simulink subsystem "Speed_PI_D"  (R2022b)
settings: Solver=VariableStepAuto  StartTime=0.0  StopTime=10.0  RelTol=1e-3
undefined symbols (not defined in the file or in its folder): conv, DiscIntNeverNeededParam, motor, Ri, Rw, sat, uc
settings Model: Creator=gotta  LastModifiedBy=gotta

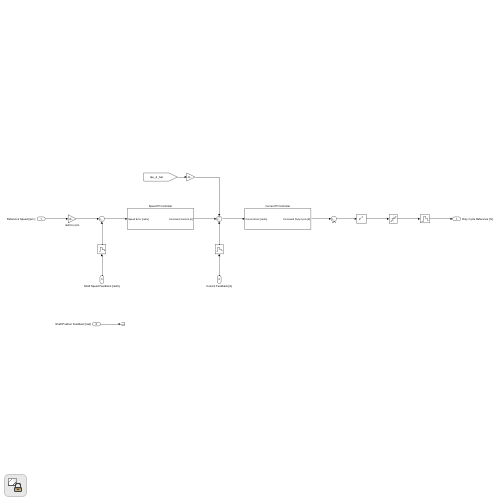
[thumbnail: Simulink's stored preview of the top-level diagram]
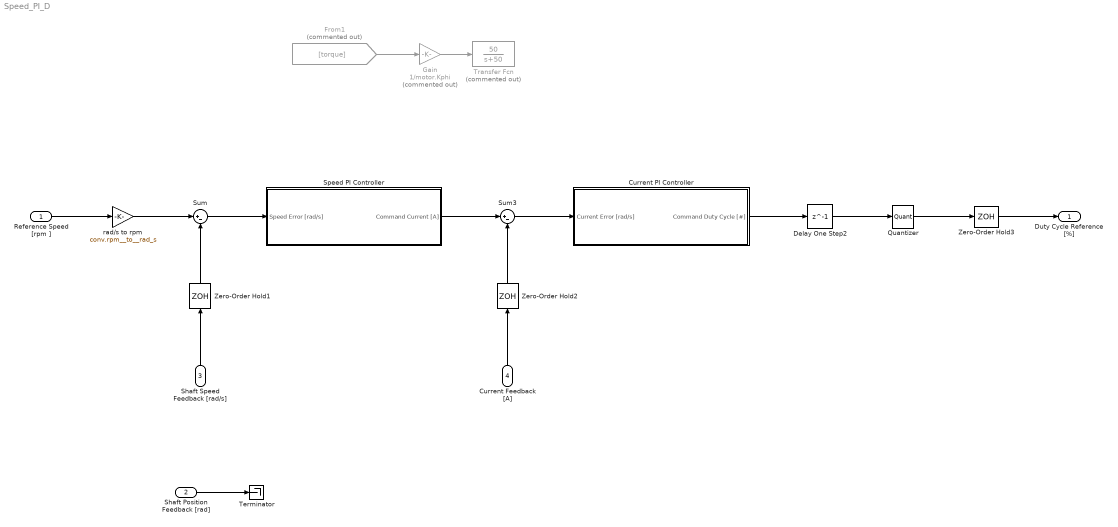
== system Speed_PI_D ==
  Reference Speed [rpm ] : Inport
  Shaft Position Feedback [rad] : Inport  Port=2
  Shaft Speed Feedback [rad/s] : Inport  Port=3
  Current Feedback [A] : Inport  Port=4
  Current PI Controller : Subsystem
  Delay One Step2 : Delay  DelayLength=1
  From1 : From  Commented=on  GotoTag=torque
  Gain : Gain  Commented=on  Gain=1/motor.Kphi
  Quantizer : Quantizer  QuantizationInterval=uc.d_step
  Speed PI Controller : Subsystem
  Sum : Sum  Inputs=|+-
  Sum3 : Sum  Inputs=|+-
  Terminator : Terminator
  Transfer Fcn : TransferFcn  Commented=on  Numerator=[50]  Denominator=[1 50]
  Zero-Order Hold1 : ZeroOrderHold  SampleTime=uc.Ts
  Zero-Order Hold2 : ZeroOrderHold  SampleTime=uc.Ts
  Zero-Order Hold3 : ZeroOrderHold  SampleTime=uc.Ts
  rad/s to rpm : Gain  Gain=conv.rpm__to__rad_s
  Duty Cycle Reference [%] : Outport
  wires:
  Shaft Speed Feedback [rad/s]/1 -> Zero-Order Hold1/1
  Delay One Step2/1 -> Quantizer/1
  Reference Speed [rpm ]/1 -> rad/s to rpm/1
  Quantizer/1 -> Zero-Order Hold3/1
  Zero-Order Hold1/1 -> Sum/2
  rad/s to rpm/1 -> Sum/1
  Zero-Order Hold3/1 -> Duty Cycle Reference [%]/1
  Shaft Position Feedback [rad]/1 -> Terminator/1
  Current Feedback [A]/1 -> Zero-Order Hold2/1
  Current PI Controller/1(Command Duty Cycle [#]) -> Delay One Step2/1
  Sum/1 -> Speed PI Controller/1(Speed Error [rad/s])
  Speed PI Controller/1(Command Current [A]) -> Sum3/1
  Sum3/1 -> Current PI Controller/1(Current Error [rad/s])
  Zero-Order Hold2/1 -> Sum3/2
  From1/1 -> Gain/1
  Gain/1 -> Transfer Fcn/1

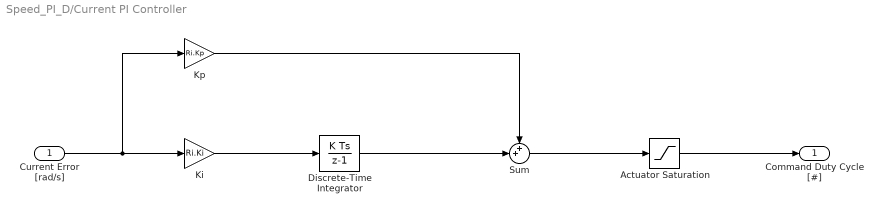
== system Speed_PI_D/Current PI Controller ==
  Current Error [rad/s] : Inport
  Actuator Saturation : Saturate  UpperLimit=sat.d  LowerLimit=-sat.d
  Discrete-Time Integrator : DiscreteIntegrator  SampleTime=uc.Ts  LimitOutput=on  UpperSaturationLimit=sat.d  LowerSaturationLimit=-sat.d  ICPrevOutput=DiscIntNeverNeededParam  ICPrevScaledInput=DiscIntNeverNeededParam
  Ki : Gain  Gain=Ri.Ki
  Kp : Gain  Gain=Ri.Kp
  Sum : Sum  Inputs=++|
  Command Duty Cycle [#] : Outport
  wires:
  Discrete-Time Integrator/1 -> Sum/2
  Ki/1 -> Discrete-Time Integrator/1
  Sum/1 -> Actuator Saturation/1
  Kp/1 -> Sum/1
  Current Error [rad/s]/1 -> Ki/1, Kp/1
  Actuator Saturation/1 -> Command Duty Cycle [#]/1

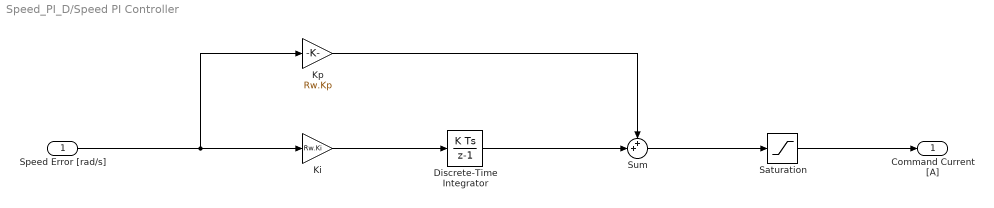
== system Speed_PI_D/Speed PI Controller ==
  Speed Error [rad/s] : Inport
  Discrete-Time Integrator : DiscreteIntegrator  SampleTime=uc.Ts  LimitOutput=on  UpperSaturationLimit=sat.I  LowerSaturationLimit=-sat.I  ICPrevOutput=DiscIntNeverNeededParam  ICPrevScaledInput=DiscIntNeverNeededParam
  Ki : Gain  Gain=Rw.Ki
  Kp : Gain  Gain=Rw.Kp
  Saturation : Saturate  UpperLimit=sat.I  LowerLimit=-sat.I
  Sum : Sum  Inputs=++|
  Command Current [A] : Outport
  wires:
  Kp/1 -> Sum/1
  Saturation/1 -> Command Current [A]/1
  Sum/1 -> Saturation/1
  Ki/1 -> Discrete-Time Integrator/1
  Discrete-Time Integrator/1 -> Sum/2
  Speed Error [rad/s]/1 -> Kp/1, Ki/1
